simulink model "uwb_6_delay_mult_optim_r2024b"  (R2024b)
settings: Solver=VariableStepAuto  StartTime=0.0  StopTime=1e-6  RelTol=1e-3
undefined symbols (not defined in the file or in its folder): j
libraries: commrfcorlib x1, commchan3 x1, commdigbbndpm3 x1, dspstat3 x1
settings Model: Creator=IWMAI  LastModifiedBy=IWMAI

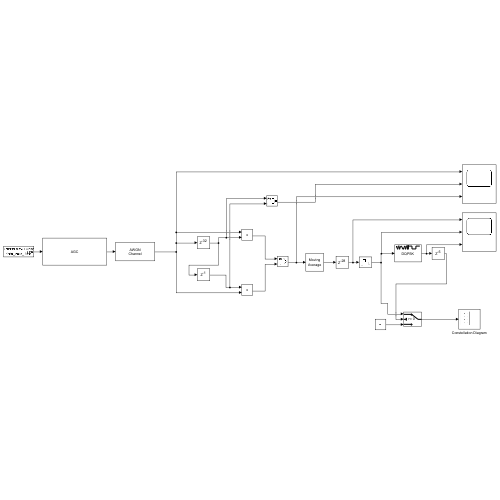
[thumbnail: Simulink's stored preview of the top-level diagram]
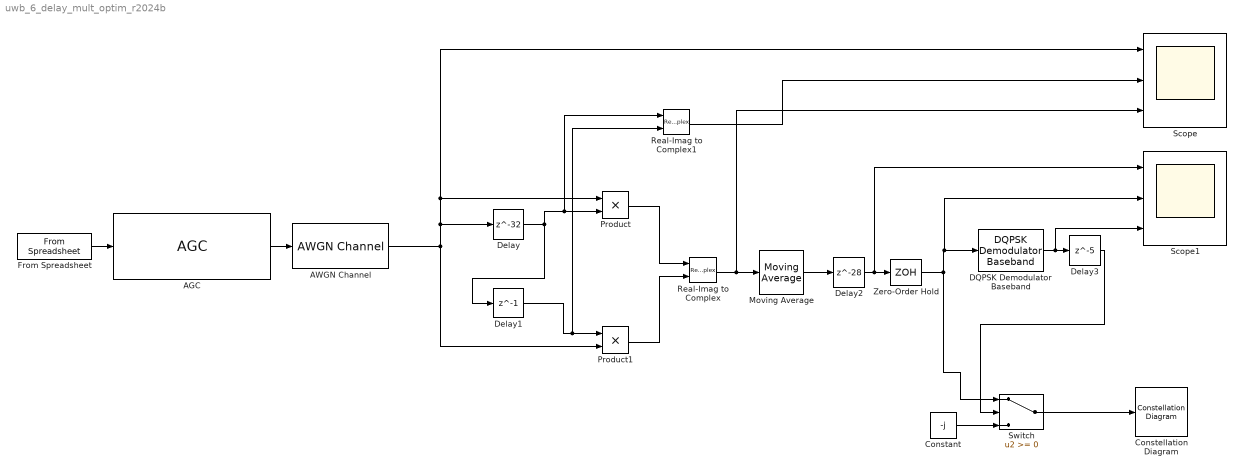
== system uwb_6_delay_mult_optim_r2024b ==
  AGC : commrfcorlib/AGC  LegacyMode=off  DetectorMethod=Rectifier  LoopMethod=Linear  UpdatePeriod=100  StepSize=0.1  AdaptationStepSize=0.01  DesiredOutputPower=1/2  AveragingLength=64  MaximumGain=30  MaxPowerGain=60  GainOutputPort=off  InputPowerOutputPort=off  SimulateUsing=Interpreted execution
  AWGN Channel : commchan3/AWGN Channel  LegacyMode=off  NoiseMethod="Signal to noise ratio  (SNR)"  noiseMode="Signal to noise ratio  (SNR)"  EbNo=10  EsNo=10  SNR=15  BitsPerSymbol=1  SignalPower=1  SamplesPerSymbol=1  SymbolPeriod=1  VarianceSource=Parameter  Variance=1  RandomStream=Global stream  Seed=67  SimulateUsing=Code generation
  Constant : Constant  Value=-j
  Constellation Diagram : ConstellationDiagram  WindowPosition=[392.000000,143.000000,790.000000,600.000000,]  ScopeFrameLocation=window  SymbolsToDisplaySource=Property  SymbolsToDisplay=2500  XLimits=[-1.47,1.47]  YLimits=[-1.38,1.38]  EnableMeasurements=on  DefaultConfigurationName=comm.scopes.ConstellationDiagramBlockCfg
  DQPSK Demodulator Baseband : commdigbbndpm3/DQPSK Demodulator Baseband  OutType=Integer  Dec=Gray  Ph=0  outDtype1=Inherit via internal rule  outDtype2=Inherit via internal rule
  Delay : Delay  DelayLength=32
  Delay1 : Delay  DelayLength=1
  Delay2 : Delay  DelayLength=28
  Delay3 : Delay  DelayLength=5
  From Spreadsheet : FromSpreadsheet  FileName=C:\Users\IWMAI\University of Toronto\Yu Huang - Summer-2025-sharted\Yongkang\v3_250617\csv\data_zero_time.csv  SheetName=data_zero_time  SampleTime=1/16e9
  Moving Average : dspstat3/Moving Average  Method=Sliding window  ForgettingFactorPort=off  SpecifyWindowLength=on  WindowLength=8  OverlapLength=7  AllowArbitraryInputLength=off  ForgettingFactor=0.9  SimulateUsing=Interpreted execution
  Product : Product
  Product1 : Product
  Real-Imag to Complex : RealImagToComplex
  Real-Imag to Complex1 : RealImagToComplex
  Scope : Scope  NumInputPorts=3
  Scope1 : Scope  NumInputPorts=3
  Switch : Switch  SaturateOnIntegerOverflow=off  InputSameDT=off
  Zero-Order Hold : ZeroOrderHold  SampleTime=1/500e6
  wires:
  From Spreadsheet/1 -> AGC/1
  AGC/1 -> AWGN Channel/1
  Delay/1 -> Delay1/1, Real-Imag to Complex1/1, Product/2
  AWGN Channel/1 -> Product1/2, Scope/1, Product/1, Delay/1
  Product/1 -> Real-Imag to Complex/1
  Product1/1 -> Real-Imag to Complex/2
  Delay1/1 -> Real-Imag to Complex1/2, Product1/1
  Real-Imag to Complex/1 -> Scope/3, Moving Average/1
  Delay2/1 -> Scope1/1, Zero-Order Hold/1
  Zero-Order Hold/1 -> Switch/1, Scope1/2, DQPSK Demodulator Baseband/1
  DQPSK Demodulator Baseband/1 -> Scope1/3, Delay3/1
  Delay3/1 -> Switch/2
  Constant/1 -> Switch/3
  Switch/1 -> Constellation Diagram/1
  Moving Average/1 -> Delay2/1
  Real-Imag to Complex1/1 -> Scope/2
